simulink model "mutant4"  (R2013b)
settings: Solver=FixedStepDiscrete  StartTime=0.0  StopTime=50  FixedStep=0.01  RelTol=1e-3
values from neighbouring files (symbols this model uses):
  IC_ALTS = S(is,3)    [code_sim.m]    (also in code_test.m)
  IC_ALTSARM = (S(is,3)==2)    [code_sim.m]    (also in code_test.m)
  IC_ALTSCAP = (S(is,3)==3)    [code_sim.m]    (also in code_test.m)
  IC_AP = S(is,2)    [code_sim.m]    (also in code_test.m)
  IC_APON = (S(is,2)==1)    [code_sim.m]    (also in code_test.m)
  IC_VERT = S(is,1)    [code_sim.m]    (also in code_test.m)
undefined symbols (not defined in the file or in its folder): sldvsubsys
libraries: sldvlib x36, simulink x21
settings Model: Creator=JYOGANAN  LastModifiedBy=Mamatha
settings DataIOCC: SignalLoggingSaveFormat=ModelDataLogs
settings DebuggingCC: MultiTaskDSMMsg=warning  MultiTaskCondExecSysMsg=none
settings RTWCC: IncludeERTFirstTime=on
settings GRTTargetCC: CodeReplacementLibrary=None  CPPClassGenCompliant=on
settings ConfigComp: Description=Design Verifier Custom Configuration Component  DVMaxProcessTime=14400  DVMaxTestCaseSteps=500  DVTestSuiteOptimization=CombinedObjectives (Nonlinear Extended)

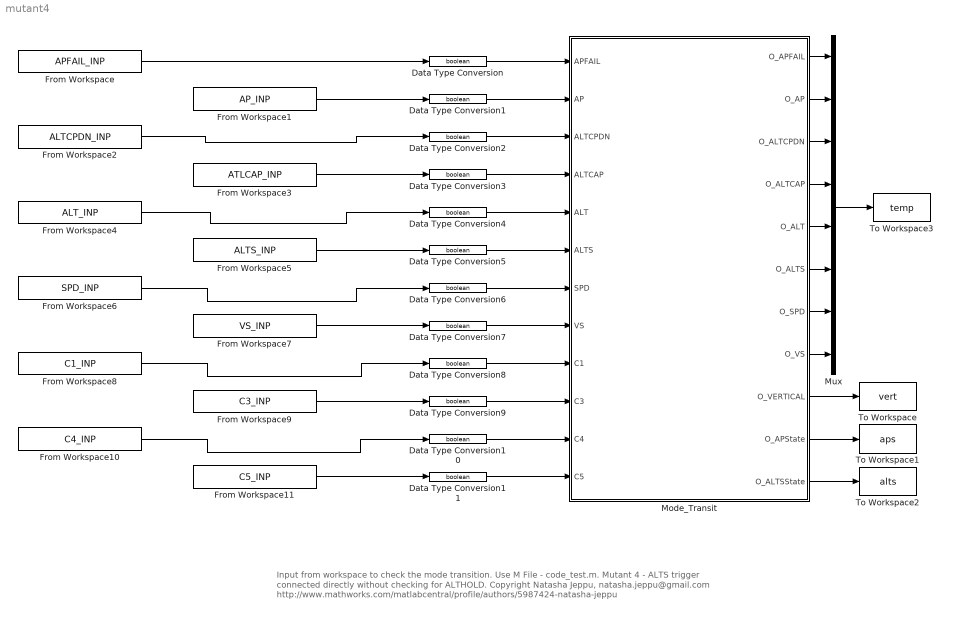
== system mutant4 ==
  note: Input from workspace to check the mode transition. Use M File - code_test.m.
      | Mutant 4 - ALTS trigger connected directly without checking for ALTHOLD.
      |
      | Copyright Natasha Jeppu, natasha.jeppu@gmail.com
      | http://www.mathworks.com/matlabcentral/profile/authors/5987424-natasha-jeppu
  Data Type Conversion{,1..11} (12 alike) : DataTypeConversion  OutDataTypeStr=boolean
  From Workspace : FromWorkspace  VariableName=APFAIL_INP  Interpolate=off  OutputAfterFinalValue=Holding final value
  From Workspace1 : FromWorkspace  VariableName=AP_INP  Interpolate=off  OutputAfterFinalValue=Holding final value
  From Workspace10 : FromWorkspace  VariableName=C4_INP  Interpolate=off  OutputAfterFinalValue=Holding final value
  From Workspace11 : FromWorkspace  VariableName=C5_INP  Interpolate=off  OutputAfterFinalValue=Holding final value
  From Workspace2 : FromWorkspace  VariableName=ALTCPDN_INP  Interpolate=off  OutputAfterFinalValue=Holding final value
  From Workspace3 : FromWorkspace  VariableName=ATLCAP_INP  Interpolate=off  OutputAfterFinalValue=Holding final value
  From Workspace4 : FromWorkspace  VariableName=ALT_INP  Interpolate=off  OutputAfterFinalValue=Holding final value
  From Workspace5 : FromWorkspace  VariableName=ALTS_INP  Interpolate=off  OutputAfterFinalValue=Holding final value
  From Workspace6 : FromWorkspace  VariableName=SPD_INP  Interpolate=off  OutputAfterFinalValue=Holding final value
  From Workspace7 : FromWorkspace  VariableName=VS_INP  Interpolate=off  OutputAfterFinalValue=Holding final value
  From Workspace8 : FromWorkspace  VariableName=C1_INP  Interpolate=off  OutputAfterFinalValue=Holding final value
  From Workspace9 : FromWorkspace  VariableName=C3_INP  Interpolate=off  OutputAfterFinalValue=Holding final value
  Mode_Transit : Subsystem
  Mux : Mux  Inputs=8
  To Workspace : ToWorkspace  VariableName=vert  SampleTime=-1
  To Workspace1 : ToWorkspace  VariableName=aps  SampleTime=-1
  To Workspace2 : ToWorkspace  VariableName=alts  SampleTime=-1
  To Workspace3 : ToWorkspace  VariableName=temp  SampleTime=-1
  wires:
  From Workspace/1 -> Data Type Conversion/1
  Mode_Transit/9(O_VERTICAL) -> To Workspace/1
  Mode_Transit/10(O_APState) -> To Workspace1/1
  Mode_Transit/11(O_ALTSState) -> To Workspace2/1
  Data Type Conversion/1 -> Mode_Transit/1(APFAIL)
  Data Type Conversion1/1 -> Mode_Transit/2(AP)
  Data Type Conversion2/1 -> Mode_Transit/3(ALTCPDN)
  Data Type Conversion3/1 -> Mode_Transit/4(ALTCAP)
  Data Type Conversion4/1 -> Mode_Transit/5(ALT)
  Data Type Conversion5/1 -> Mode_Transit/6(ALTS)
  Data Type Conversion6/1 -> Mode_Transit/7(SPD)
  Data Type Conversion7/1 -> Mode_Transit/8(VS)
  Data Type Conversion8/1 -> Mode_Transit/9(C1)
  Data Type Conversion9/1 -> Mode_Transit/10(C3)
  Data Type Conversion10/1 -> Mode_Transit/11(C4)
  Data Type Conversion11/1 -> Mode_Transit/12(C5)
  From Workspace1/1 -> Data Type Conversion1/1
  From Workspace2/1 -> Data Type Conversion2/1
  From Workspace3/1 -> Data Type Conversion3/1
  From Workspace4/1 -> Data Type Conversion4/1
  From Workspace5/1 -> Data Type Conversion5/1
  From Workspace6/1 -> Data Type Conversion6/1
  From Workspace7/1 -> Data Type Conversion7/1
  From Workspace8/1 -> Data Type Conversion8/1
  From Workspace9/1 -> Data Type Conversion9/1
  From Workspace10/1 -> Data Type Conversion10/1
  From Workspace11/1 -> Data Type Conversion11/1
  Mux/1 -> To Workspace3/1
  Mode_Transit/3(O_ALTCPDN) -> Mux/3
  Mode_Transit/4(O_ALTCAP) -> Mux/4
  Mode_Transit/2(O_AP) -> Mux/2
  Mode_Transit/5(O_ALT) -> Mux/5
  Mode_Transit/1(O_APFAIL) -> Mux/1
  Mode_Transit/6(O_ALTS) -> Mux/6
  Mode_Transit/7(O_SPD) -> Mux/7
  Mode_Transit/8(O_VS) -> Mux/8

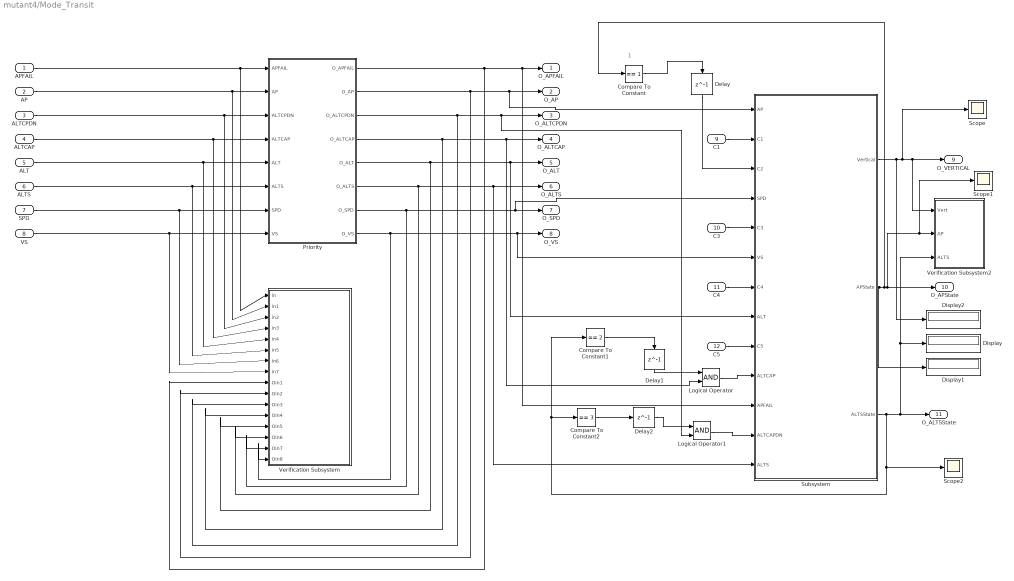
== system mutant4/Mode_Transit ==
  note: 1
  APFAIL : Inport
  AP : Inport  Port=2
  ALTCPDN : Inport  Port=3
  ALTCAP : Inport  Port=4
  ALT : Inport  Port=5
  ALTS : Inport  Port=6
  SPD : Inport  Port=7
  VS : Inport  Port=8
  C1 : Inport  Port=9
  C3 : Inport  Port=10
  C4 : Inport  Port=11
  C5 : Inport  Port=12
  Compare To Constant : simulink/Logic and Bit Operations/Compare To Constant  relop===  const=1  OutDataTypeStr=boolean
  Compare To Constant1 : simulink/Logic and Bit Operations/Compare To Constant  relop===  const=2  OutDataTypeStr=boolean
  Compare To Constant2 : simulink/Logic and Bit Operations/Compare To Constant  relop===  const=3  OutDataTypeStr=boolean
  Delay : Delay  DelayLength=1  InitialCondition=IC_APON
  Delay1 : Delay  DelayLength=1  InitialCondition=IC_ALTSARM
  Delay2 : Delay  DelayLength=1  InitialCondition=IC_ALTSCAP
  Display : Display
  Display1 : Display
  Display2 : Display
  Logical Operator : Logic  AllPortsSameDT=off  OutDataTypeStr=boolean
  Logical Operator1 : Logic  AllPortsSameDT=off  OutDataTypeStr=boolean
  Priority : Subsystem
  Scope : Scope
  Scope1 : Scope
  Scope2 : Scope
      settings: SaveName=ScopeData2
  Subsystem : Subsystem
  Verification Subsystem : Subsystem  Tag=VerificationSubsystem  DisableCoverage=on  LoadFcn=sldvsubsys('check')  TreatAsAtomicUnit=on  SimViewingDevice=on  mask(VerificationSubsystem){}
      mask init:
      | sldvsubsys('maskInit');
      settings: CopyFcn=sldvsubsys('copy');  OpenFcn=open_system(gcb,'force');
      settings: PreSaveFcn=|
      | set_param(gcb,'SimViewingDevice','on');
      | sldvsubsys('check');
      mask Help: helpview(fullfile(docroot,'toolbox','sldv','sldv.map'),'verificationsubsystem')
      mask Display: image(imread('sldvicon_versubsys.png','BackGroundColor',[1 1 1]),'center');
  Verification Subsystem2 : Subsystem  Tag=VerificationSubsystem  DisableCoverage=on  LoadFcn=sldvsubsys('check')  TreatAsAtomicUnit=on  SimViewingDevice=on  mask(VerificationSubsystem){}
      mask init:
      | sldvsubsys('maskInit');
      settings: CopyFcn=sldvsubsys('copy');  OpenFcn=open_system(gcb,'force');
      settings: PreSaveFcn=|
      | set_param(gcb,'SimViewingDevice','on');
      | sldvsubsys('check');
      mask Help: helpview(fullfile(docroot,'toolbox','sldv','sldv.map'),'verificationsubsystem')
      mask Display: image(imread('sldvicon_versubsys.png','BackGroundColor',[1 1 1]),'center');
  O_APFAIL : Outport
  O_AP : Outport  Port=2
  O_ALTCPDN : Outport  Port=3
  O_ALTCAP : Outport  Port=4
  O_ALT : Outport  Port=5
  O_ALTS : Outport  Port=6
  O_SPD : Outport  Port=7
  O_VS : Outport  Port=8
  O_VERTICAL : Outport  Port=9
  O_APState : Outport  Port=10
  O_ALTSState : Outport  Port=11
  wires:
  Priority/2(O_AP) -> Verification Subsystem/10(Oin2), O_AP/1, Subsystem/1(AP)
  Priority/3(O_ALTCPDN) -> Verification Subsystem/11(Oin3), Logical Operator1/2, O_ALTCPDN/1
  Priority/1(O_APFAIL) -> Verification Subsystem/9(Oin1), O_APFAIL/1, Subsystem/11(APFAIL)
  Priority/4(O_ALTCAP) -> Verification Subsystem/12(Oin4), O_ALTCAP/1, Logical Operator/2
  Priority/6(O_ALTS) -> Verification Subsystem/14(Oin6), Subsystem/13(ALTS), O_ALTS/1
  Priority/8(O_VS) -> Verification Subsystem/16(Oin8), O_VS/1, Subsystem/6(VS)
  ALT/1 -> Verification Subsystem/5(in4), Priority/5(ALT)
  APFAIL/1 -> Verification Subsystem/1(in), Priority/1(APFAIL)
  AP/1 -> Verification Subsystem/2(in1), Priority/2(AP)
  ALTCAP/1 -> Verification Subsystem/4(in3), Priority/4(ALTCAP)
  ALTS/1 -> Verification Subsystem/6(in5), Priority/6(ALTS)
  SPD/1 -> Verification Subsystem/7(in6), Priority/7(SPD)
  VS/1 -> Verification Subsystem/8(in7), Priority/8(VS)
  ALTCPDN/1 -> Verification Subsystem/3(in2), Priority/3(ALTCPDN)
  Priority/7(O_SPD) -> Verification Subsystem/15(Oin7), O_SPD/1, Subsystem/4(SPD)
  Priority/5(O_ALT) -> Verification Subsystem/13(Oin5), O_ALT/1, Subsystem/8(ALT)
  C1/1 -> Subsystem/2(C1)
  Compare To Constant/1 -> Delay/1
  C3/1 -> Subsystem/5(C3)
  C4/1 -> Subsystem/7(C4)
  C5/1 -> Subsystem/9(C5)
  Subsystem/1(Vertical) -> Display2/1, Scope/1, Verification Subsystem2/1(Vert), O_VERTICAL/1
  Delay/1 -> Subsystem/3(C2)
  Compare To Constant1/1 -> Delay1/1
  Delay1/1 -> Logical Operator/1
  Delay2/1 -> Logical Operator1/1
  Compare To Constant2/1 -> Delay2/1
  Subsystem/2(APState) -> Compare To Constant/1, O_APState/1, Verification Subsystem2/2(AP), Scope1/1, Display1/1
  Subsystem/3(ALTSState) -> Scope2/1, Compare To Constant2/1, Compare To Constant1/1, O_ALTSState/1, Verification Subsystem2/3(ALTS), Display/1
  Logical Operator/1 -> Subsystem/10(ALTCAP)
  Logical Operator1/1 -> Subsystem/12(ALTCAPDN)

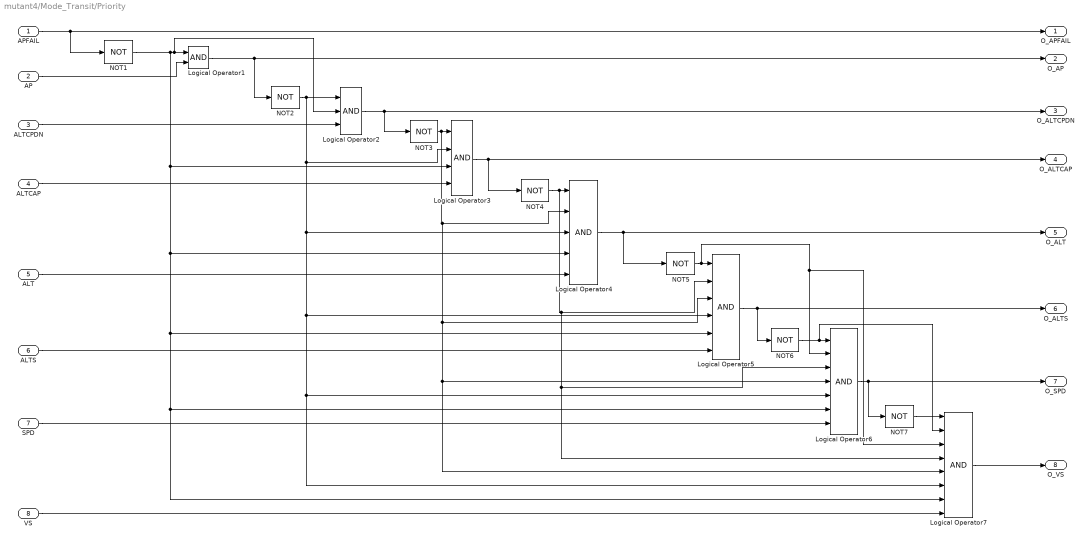
== system mutant4/Mode_Transit/Priority ==
  APFAIL : Inport
  AP : Inport  Port=2
  ALTCPDN : Inport  Port=3
  ALTCAP : Inport  Port=4
  ALT : Inport  Port=5
  ALTS : Inport  Port=6
  SPD : Inport  Port=7
  VS : Inport  Port=8
  Logical Operator1 : Logic  AllPortsSameDT=off  OutDataTypeStr=boolean
  Logical Operator2 : Logic  Inputs=3  AllPortsSameDT=off  OutDataTypeStr=boolean
  Logical Operator3 : Logic  Inputs=4  AllPortsSameDT=off  OutDataTypeStr=boolean
  Logical Operator4 : Logic  Inputs=5  AllPortsSameDT=off  OutDataTypeStr=boolean
  Logical Operator5 : Logic  Inputs=6  AllPortsSameDT=off  OutDataTypeStr=boolean
  Logical Operator6 : Logic  Inputs=7  AllPortsSameDT=off  OutDataTypeStr=boolean
  Logical Operator7 : Logic  Inputs=8  AllPortsSameDT=off  OutDataTypeStr=boolean
  NOT{1..7} (7 alike) : Logic  Operator=NOT  AllPortsSameDT=off  OutDataTypeStr=boolean
  O_APFAIL : Outport
  O_AP : Outport  Port=2
  O_ALTCPDN : Outport  Port=3
  O_ALTCAP : Outport  Port=4
  O_ALT : Outport  Port=5
  O_ALTS : Outport  Port=6
  O_SPD : Outport  Port=7
  O_VS : Outport  Port=8
  wires:
  AP/1 -> Logical Operator1/2
  APFAIL/1 -> O_APFAIL/1, NOT1/1
  NOT1/1 -> Logical Operator2/2, Logical Operator1/1, Logical Operator3/3, Logical Operator4/4, Logical Operator5/5, Logical Operator6/6, Logical Operator7/7
  Logical Operator1/1 -> NOT2/1, O_AP/1
  ALTCPDN/1 -> Logical Operator2/3
  NOT2/1 -> Logical Operator7/6, Logical Operator6/5, Logical Operator5/4, Logical Operator4/3, Logical Operator3/2, Logical Operator2/1
  Logical Operator2/1 -> NOT3/1, O_ALTCPDN/1
  ALTCAP/1 -> Logical Operator3/4
  NOT3/1 -> Logical Operator7/5, Logical Operator6/4, Logical Operator5/3, Logical Operator4/2, Logical Operator3/1
  Logical Operator3/1 -> NOT4/1, O_ALTCAP/1
  NOT4/1 -> Logical Operator7/4, Logical Operator6/3, Logical Operator5/2, Logical Operator4/1
  ALT/1 -> Logical Operator4/5
  Logical Operator4/1 -> NOT5/1, O_ALT/1
  NOT5/1 -> Logical Operator7/3, Logical Operator6/2, Logical Operator5/1
  ALTS/1 -> Logical Operator5/6
  Logical Operator5/1 -> NOT6/1, O_ALTS/1
  NOT6/1 -> Logical Operator7/2, Logical Operator6/1
  SPD/1 -> Logical Operator6/7
  NOT7/1 -> Logical Operator7/1
  Logical Operator6/1 -> NOT7/1, O_SPD/1
  VS/1 -> Logical Operator7/8
  Logical Operator7/1 -> O_VS/1

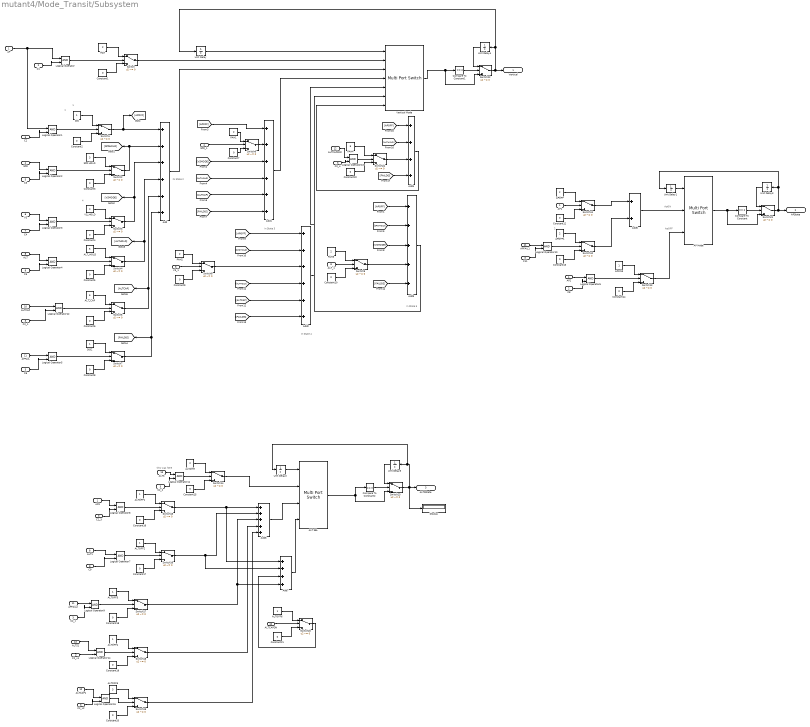
== system mutant4/Mode_Transit/Subsystem ==
  note: this was here
  note: 2
  note: 1
  note: 4
  note: 1
  note: In State 5
  note: In State 4
  note: In State 3
  note: IN State 2
  note: ApON
  note: ApOFF
  AP : Inport
  C1 : Inport  Port=2
  C2 : Inport  Port=3
  SPD : Inport  Port=4
  C3 : Inport  Port=5
  VS : Inport  Port=6
  C4 : Inport  Port=7
  ALT : Inport  Port=8
  C5 : Inport  Port=9
  ALTCAP : Inport  Port=10
  APFAIL : Inport  Port=11
  ALTCAPDN : Inport  Port=12
  ALTS : Inport  Port=13
  ALT SEL : MultiPortSwitch
  ALT1 : InportShadow  Port=8
  ALTARM : Constant  Value=2
  ALTCAP1 : InportShadow  Port=10
  ALTCAPDN2 : InportShadow  Port=12
  ALTOFF{1..4,6} (5 alike) : Constant
  ALTOFF5 : Constant  Value=3
  ALTS1 : InportShadow  Port=13
  ALT_1 : InportShadow  Port=8
  ALT_CAP : Constant  Value=6
  ALT_HOLD : Constant  Value=5
  AP Mode : MultiPortSwitch  Inputs=2
  AP1 : InportShadow
  AP2 : InportShadow
  AP3 : InportShadow
  APFAIL1 : InportShadow  Port=11
  APFAIL2 : InportShadow  Port=11
  APOFF : Constant  Value=2
  APOFF1 : Constant  Value=2
  APON3 : Constant
  Add : Sum  Inputs=++++++
  Add1 : Sum  Inputs=++++++
  Add2 : Sum  Inputs=++++++
  Add3 : Sum  Inputs=+++++
  Add4 : Sum  Inputs=++++
  Add5 : Sum
  Add6 : Sum  Inputs=+++++
  Add7 : Sum  Inputs=++++
  C11 : InportShadow  Port=3
  C2_{1..4} (4 alike) : InportShadow  Port=3
  C2_x : InportShadow  Port=3
  C2_x1 : InportShadow  Port=3
  C2_x2 : InportShadow  Port=3
  C6 : InportShadow  Port=3
  C8 : InportShadow  Port=2
  C9 : InportShadow  Port=9
  Compare To Constant : simulink/Logic and Bit Operations/Compare To Constant  relop===  const=0  OutDataTypeStr=boolean
  Compare To Constant1 : simulink/Logic and Bit Operations/Compare To Constant  relop===  const=0  OutDataTypeStr=boolean
  Compare To Constant2 : simulink/Logic and Bit Operations/Compare To Constant  relop===  const=0  OutDataTypeStr=boolean
  Constant{1..10,12..22} (21 alike) : Constant  Value=0
  DIS : Constant
  DISC : Constant
  Display : Display
  Logical Operator{,1..15} (16 alike) : Logic  IconShape=distinctive  AllPortsSameDT=off  OutDataTypeStr=boolean
  PAH{,1..3} (4 alike) : Constant  Value=2
  PAH4 : Constant  Value=5
  SPD HOLD : Constant  Value=3
  SPD_1 : InportShadow  Port=4
  Switch{,1..9,11..24} (24 alike) : Switch  Criteria=u2 ~= 0
  Unit Delay : UnitDelay  InitialCondition=IC_VERT  SampleTime=-1
  Unit Delay1 : UnitDelay  InitialCondition=IC_AP  SampleTime=-1
  Unit Delay2 : UnitDelay  InitialCondition=IC_ALTS  SampleTime=-1
  Unit Delay3 : UnitDelay  InitialCondition=IC_AP  SampleTime=-1
  Unit Delay4 : UnitDelay  InitialCondition=IC_VERT  SampleTime=-1
  Unit Delay5 : UnitDelay  InitialCondition=IC_ALTS  SampleTime=-1
  VS_1 : InportShadow  Port=6
  VS_HOLD : Constant  Value=4
  Vertical Mode : MultiPortSwitch  Inputs=6
  Vertical : Outport
  APState : Outport  Port=2
  ALTSState : Outport  Port=3
  wires:
  Unit Delay/1 -> Vertical Mode/1
  PAH/1 -> Switch/1
  Constant1/1 -> Switch/3
  C1/1 -> Logical Operator/2
  Logical Operator/1 -> Switch/2
  Switch/1 -> Vertical Mode/2
  DIS/1 -> Switch1/1
  Constant2/1 -> Switch1/3
  AP/1 -> Logical Operator1/1, Logical Operator/1
  C2/1 -> Logical Operator1/2
  Logical Operator1/1 -> Switch1/2
  SPD HOLD/1 -> Switch2/1
  Constant3/1 -> Switch2/3
  SPD/1 -> Logical Operator2/1
  C3/1 -> Logical Operator2/2
  Logical Operator2/1 -> Switch2/2
  Switch2/1 -> [SPDHOLD], Add/2
  Add/1 -> Vertical Mode/3
  Constant8/1 -> Switch7/3
  DISC/1 -> Switch7/1
  Switch3/1 -> Add/3, [VSMODE]
  Logical Operator3/1 -> Switch3/2
  C4/1 -> Logical Operator3/2
  VS/1 -> Logical Operator3/1
  Constant4/1 -> Switch3/3
  VS_HOLD/1 -> Switch3/1
  C5/1 -> Logical Operator4/2
  Logical Operator4/1 -> Switch4/2
  ALT_HOLD/1 -> Switch4/1
  Constant5/1 -> Switch4/3
  ALT/1 -> Logical Operator4/1
  ALT_CAP/1 -> Switch5/1
  Constant6/1 -> Switch5/3
  ALT_1/1 -> Switch9/2
  Constant10/1 -> Switch9/3
  Switch9/1 -> Add3/4
  PAH3/1 -> Switch9/1
  Switch5/1 -> [ALTCAP], Add/5
  SPD_1/1 -> Switch6/2
  Constant7/1 -> Switch6/3
  Switch4/1 -> [ALTHOLD], Add/4
  PAH1/1 -> Switch6/1
  Constant9/1 -> Switch8/3
  PAH2/1 -> Switch8/1
  VS_1/1 -> Switch8/2
  APFAIL/1 -> Logical Operator5/1
  Logical Operator5/1 -> Switch7/2
  C6/1 -> Logical Operator5/2
  Unit Delay1/1 -> AP Mode/1
  Constant12/1 -> Switch11/3
  APOFF/1 -> Switch11/1
  Switch11/1 -> Add5/1
  Constant13/1 -> Switch12/3
  APOFF1/1 -> Switch12/1
  Switch12/1 -> Add5/2
  Constant14/1 -> Switch13/3
  APON3/1 -> Switch13/1
  AP1/1 -> Switch11/2
  C8/1 -> Logical Operator6/2
  Add5/1 -> AP Mode/2
  Switch13/1 -> AP Mode/3
  Logical Operator6/1 -> Switch13/2
  AP2/1 -> Logical Operator6/1
  Unit Delay2/1 -> ALT SEL/1
  Constant15/1 -> Switch14/3
  ALTARM/1 -> Switch14/1
  Constant16/1 -> Switch15/3
  ALTOFF1/1 -> Switch15/1
  Switch15/1 -> Add7/1, Add6/1
  Logical Operator8/1 -> Switch15/2
  Constant17/1 -> Switch16/3
  ALTOFF2/1 -> Switch16/1
  Switch16/1 -> Add7/2, Add6/2
  Logical Operator7/1 -> Switch16/2
  C2_3/1 -> Logical Operator8/2
  AP3/1 -> Logical Operator8/1
  ALT1/1 -> Logical Operator7/1
  C9/1 -> Logical Operator7/2
  Constant18/1 -> Switch17/3
  ALTOFF3/1 -> Switch17/1
  Switch17/1 -> Add7/4, Add6/3
  Logical Operator9/1 -> Switch17/2
  APFAIL2/1 -> Logical Operator9/1
  C2_x/1 -> Logical Operator9/2
  Constant19/1 -> Switch18/3
  ALTOFF4/1 -> Switch18/1
  Switch18/1 -> Add6/4
  Logical Operator14/1 -> Switch18/2
  Constant20/1 -> Switch19/3
  ALTOFF5/1 -> Switch19/1
  Switch19/1 -> Add6/5
  Logical Operator15/1 -> Switch19/2
  Constant21/1 -> Switch20/3
  ALTOFF6/1 -> Switch20/1
  ALTCAPDN/1 -> Switch20/2
  Switch20/1 -> Add7/3
  Logical Operator10/1 -> Switch12/2
  APFAIL1/1 -> Logical Operator10/1
  C11/1 -> Logical Operator10/2
  Switch14/1 -> ALT SEL/2
  Add6/1 -> ALT SEL/3
  Add7/1 -> ALT SEL/4
  Compare To Constant/1 -> Switch21/2
  Unit Delay3/1 -> Switch21/1
  AP Mode/1 -> Switch21/3, Compare To Constant/1
  Switch21/1 -> APState/1, Unit Delay3/1, Unit Delay1/1
  Compare To Constant1/1 -> Switch22/2
  Unit Delay4/1 -> Switch22/1
  Vertical Mode/1 -> Switch22/3, Compare To Constant1/1
  Switch22/1 -> Vertical/1, Unit Delay4/1, Unit Delay/1
  Compare To Constant2/1 -> Switch23/2
  Unit Delay5/1 -> Switch23/1
  ALT SEL/1 -> Compare To Constant2/1, Switch23/3
  Switch23/1 -> Display/1, Unit Delay2/1, Unit Delay5/1, ALTSState/1
  C2_2/1 -> Logical Operator11/2
  ALTCAP/1 -> Logical Operator12/1
  Logical Operator12/1 -> Switch5/2
  C2_1/1 -> Logical Operator12/2
  Switch7/1 -> [FAILDIS], Add/6
  Switch1/1 -> [APOFF], Add/1
  [APOFF] -> Add1/1
  [VSMODE] -> Add1/3
  [ALTHOLD] -> Add1/4
  [ALTCAP] -> Add1/5
  [FAILDIS] -> Add1/6
  Switch6/1 -> Add1/2
  Add1/1 -> Vertical Mode/4
  [APOFF] -> Add2/1
  [SPDHOLD] -> Add2/2
  Switch8/1 -> Add2/3
  [ALTHOLD] -> Add2/4
  [ALTCAP] -> Add2/5
  [FAILDIS] -> Add2/6
  Add2/1 -> Vertical Mode/5
  [APOFF] -> Add3/1
  [SPDHOLD] -> Add3/2
  [VSMODE] -> Add3/3
  [FAILDIS] -> Add3/5
  Add3/1 -> Vertical Mode/6
  Add4/1 -> Vertical Mode/7
  [APOFF] -> Add4/1
  [ALTHOLD] -> Add4/2
  Constant22/1 -> Switch24/3
  PAH4/1 -> Switch24/1
  Logical Operator13/1 -> Switch24/2
  Switch24/1 -> Add4/3
  [FAILDIS] -> Add4/4
  ALTCAPDN2/1 -> Logical Operator13/1
  C2_4/1 -> Logical Operator13/2
  ALTS1/1 -> Logical Operator14/1
  C2_x1/1 -> Logical Operator14/2
  ALTCAP1/1 -> Logical Operator15/1
  C2_x2/1 -> Logical Operator15/2
  ALTS/1 -> Logical Operator11/1
  Logical Operator11/1 -> Switch14/2

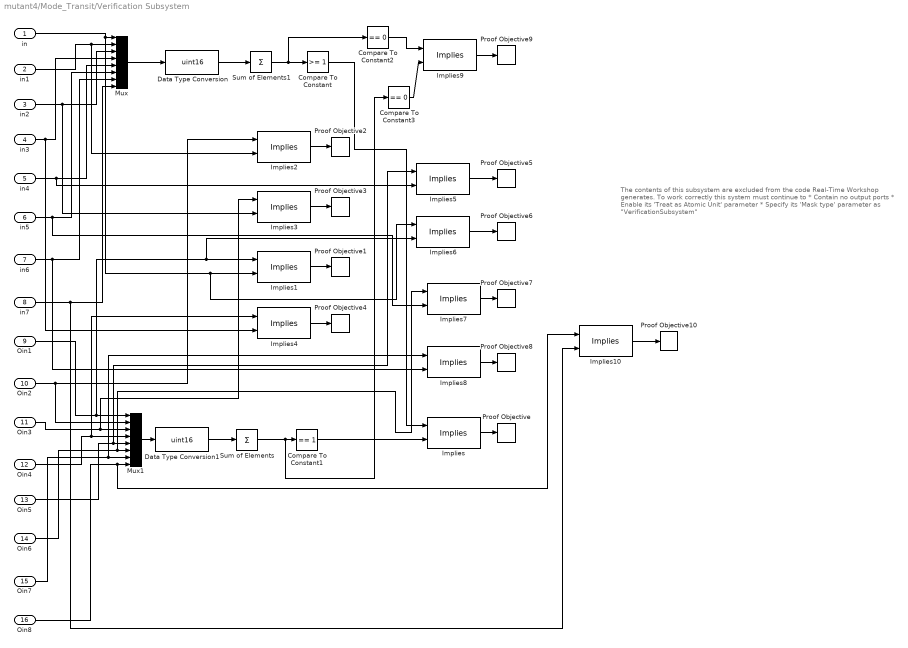
== system mutant4/Mode_Transit/Verification Subsystem ==
  note: The contents of this subsystem are excluded from the code Real-Time
      | Workshop generates.
      |
      | To work correctly this system must continue to
      | * Contain no output ports
      | * Enable its 'Treat as Atomic Unit' parameter
      | * Specify its 'Mask type' parameter as "VerificationSubsystem"
  in : Inport
  in1 : Inport  Port=2
  in2 : Inport  Port=3
  in3 : Inport  Port=4
  in4 : Inport  Port=5
  in5 : Inport  Port=6
  in6 : Inport  Port=7
  in7 : Inport  Port=8
  Oin1 : Inport  Port=9
  Oin2 : Inport  Port=10
  Oin3 : Inport  Port=11
  Oin4 : Inport  Port=12
  Oin5 : Inport  Port=13
  Oin6 : Inport  Port=14
  Oin7 : Inport  Port=15
  Oin8 : Inport  Port=16
  Compare To Constant : simulink/Logic and Bit Operations/Compare To Constant  relop=>=  const=1  OutDataTypeStr=boolean
  Compare To Constant1 : simulink/Logic and Bit Operations/Compare To Constant  relop===  const=1  OutDataTypeStr=boolean
  Compare To Constant2 : simulink/Logic and Bit Operations/Compare To Constant  relop===  const=0  OutDataTypeStr=boolean
  Compare To Constant3 : simulink/Logic and Bit Operations/Compare To Constant  relop===  const=0  OutDataTypeStr=boolean
  Data Type Conversion : DataTypeConversion  OutDataTypeStr=uint16
  Data Type Conversion1 : DataTypeConversion  OutDataTypeStr=uint16
  Implies{,1..10} (11 alike) : sldvlib/Verification Utilities/Implies
  Mux : Mux  Inputs=8
  Mux1 : Mux  Inputs=8
  Proof Objective{,1..10} (11 alike) : sldvlib/Objectives and Constraints/Proof Objective  enabled=on  customAVTBlockType=Proof Objective  intervals=true  dispValues=on  outEnabled=off  enableStopSim=off
      settings: AttributesFormatString=%<intervals>
  Sum of Elements : Sum  Inputs=+
  Sum of Elements1 : Sum  Inputs=+
  wires:
  in1/1 -> Implies2/2, Mux/2
  in2/1 -> Implies3/2, Mux/3
  in3/1 -> Implies4/2, Mux/4
  in4/1 -> Implies5/2, Mux/5
  in5/1 -> Implies7/2, Mux/6
  in6/1 -> Implies8/2, Mux/7
  in7/1 -> Implies10/2, Mux/8
  Oin1/1 -> Implies6/2, Implies1/1, Mux1/1
  Oin2/1 -> Implies2/1, Mux1/2
  Oin3/1 -> Implies3/1, Mux1/3
  Oin4/1 -> Implies4/1, Mux1/4
  Oin5/1 -> Implies5/1, Mux1/5
  Oin6/1 -> Implies7/1, Mux1/6
  Oin7/1 -> Implies8/1, Mux1/7
  Oin8/1 -> Implies10/1, Mux1/8
  Mux/1 -> Data Type Conversion/1
  Mux1/1 -> Data Type Conversion1/1
  Data Type Conversion1/1 -> Sum of Elements/1
  Data Type Conversion/1 -> Sum of Elements1/1
  Sum of Elements1/1 -> Compare To Constant2/1, Compare To Constant/1
  Sum of Elements/1 -> Compare To Constant3/1, Compare To Constant1/1
  Compare To Constant1/1 -> Implies/2
  Compare To Constant/1 -> Implies/1
  Implies/1 -> Proof Objective/1
  in/1 -> Implies6/1, Implies1/2, Mux/1
  Implies1/1 -> Proof Objective1/1
  Implies2/1 -> Proof Objective2/1
  Implies3/1 -> Proof Objective3/1
  Implies4/1 -> Proof Objective4/1
  Implies5/1 -> Proof Objective5/1
  Implies6/1 -> Proof Objective6/1
  Implies7/1 -> Proof Objective7/1
  Implies8/1 -> Proof Objective8/1
  Implies9/1 -> Proof Objective9/1
  Compare To Constant2/1 -> Implies9/1
  Compare To Constant3/1 -> Implies9/2
  Implies10/1 -> Proof Objective10/1

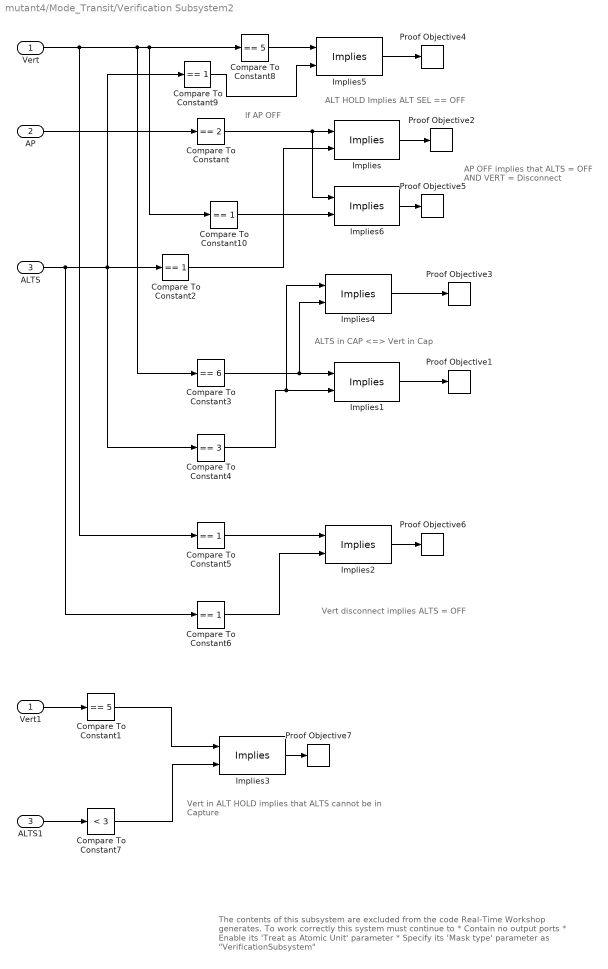
== system mutant4/Mode_Transit/Verification Subsystem2 ==
  note: ALTS in CAP <=> Vert in Cap
  note: Vert in ALT HOLD implies that ALTS cannot be
      | in Capture
  note: AP OFF implies that ALTS = OFF
      | AND VERT = Disconnect
  note: ALT HOLD Implies ALT SEL == OFF
  note: Vert disconnect implies ALTS = OFF
  note: If AP OFF
  note: The contents of this subsystem are excluded from the code Real-Time
      | Workshop generates.
      |
      | To work correctly this system must continue to
      | * Contain no output ports
      | * Enable its 'Treat as Atomic Unit' parameter
      | * Specify its 'Mask type' parameter as "VerificationSubsystem"
  Vert : Inport
  AP : Inport  Port=2
  ALTS : Inport  Port=3
  ALTS1 : InportShadow  Port=3
  Compare To Constant : simulink/Logic and Bit Operations/Compare To Constant  relop===  const=2  OutDataTypeStr=boolean
  Compare To Constant1 : simulink/Logic and Bit Operations/Compare To Constant  relop===  const=5  OutDataTypeStr=boolean
  Compare To Constant{2,5..6,9..10} (5 alike) : simulink/Logic and Bit Operations/Compare To Constant  relop===  const=1  OutDataTypeStr=boolean
  Compare To Constant3 : simulink/Logic and Bit Operations/Compare To Constant  relop===  const=6  OutDataTypeStr=boolean
  Compare To Constant4 : simulink/Logic and Bit Operations/Compare To Constant  relop===  const=3  OutDataTypeStr=boolean
  Compare To Constant7 : simulink/Logic and Bit Operations/Compare To Constant  relop=<  const=3  OutDataTypeStr=boolean
  Compare To Constant8 : simulink/Logic and Bit Operations/Compare To Constant  relop===  const=5  OutDataTypeStr=boolean
  Implies{,1..6} (7 alike) : sldvlib/Verification Utilities/Implies
  Proof Objective{1..7} (7 alike) : sldvlib/Objectives and Constraints/Proof Objective  enabled=on  customAVTBlockType=Proof Objective  intervals=true  dispValues=on  outEnabled=off  enableStopSim=on
      settings: AttributesFormatString=%<intervals>
  Vert1 : InportShadow
  wires:
  Compare To Constant/1 -> Implies6/1, Implies/1
  AP/1 -> Compare To Constant/1
  Vert/1 -> Compare To Constant5/1, Compare To Constant10/1, Compare To Constant8/1, Compare To Constant3/1
  ALTS/1 -> Compare To Constant6/1, Compare To Constant9/1, Compare To Constant4/1, Compare To Constant2/1
  Compare To Constant3/1 -> Implies4/2, Implies1/1
  Compare To Constant4/1 -> Implies4/1, Implies1/2
  Compare To Constant5/1 -> Implies2/1
  Compare To Constant6/1 -> Implies2/2
  Vert1/1 -> Compare To Constant1/1
  ALTS1/1 -> Compare To Constant7/1
  Compare To Constant1/1 -> Implies3/1
  Compare To Constant7/1 -> Implies3/2
  Compare To Constant2/1 -> Implies/2
  Implies1/1 -> Proof Objective1/1
  Implies/1 -> Proof Objective2/1
  Implies4/1 -> Proof Objective3/1
  Compare To Constant8/1 -> Implies5/1
  Implies5/1 -> Proof Objective4/1
  Compare To Constant9/1 -> Implies5/2
  Compare To Constant10/1 -> Implies6/2
  Implies6/1 -> Proof Objective5/1
  Implies2/1 -> Proof Objective6/1
  Implies3/1 -> Proof Objective7/1
